simulink model "osek_asap2"  (Simulink 6.0)
settings: Solver=FixedStepDiscrete  StartTime=0.0  StopTime=100.0  RelTol=1e-3
PreLoadFcn:
  | mysig = ASAP2.Signal;
  | mysig.RTWInfo.StorageClass = 'ExportedGlobal';
  | mysig.set('LongID_ASAP2',...
  |   'ExportedGlobal signal - unstructured data',...
  |   'PhysicalMin_ASAP2', -3, ...
  |   'PhysicalMax_ASAP2',  3, ...
  |   'Units_ASAP2',  'rpm');
  | mysig
  | myprm = ASAP2.Parameter;
  | myprm.RTWInfo.StorageClass = 'ExportedGlobal';
  | myprm.set('LongID_ASAP2',...
  |   'ExportedGlobal parameter - unstructured data',...
  |   'PhysicalMin_ASAP2', 0, ...
  |   'PhysicalMax_ASAP2', 15, ...
  |   'Value', 10, ...
  |   'Units_ASAP2',  'none');
  | myprm
settings Model: Creator=jcarrick  LastModifiedBy=jcarrick  ProdHWDeviceType=Motorola PowerPC
settings SolverCC: PositivePriorityOrder=on
settings DataIOCC: SaveOutput=off  SaveTime=off  SignalLoggingName=sigsOut
settings OptimizationCC: InlineParams=on  OptimizeModelRefInitCode=on  LifeSpan=1
settings DebuggingCC: CheckExecutionContextPreStartOutputMsg=on  CheckExecutionContextRuntimeOutputMsg=on  SolverPrmCheckMsg=none
settings HardwareCC: ProdEndianess=BigEndian  ProdHWDeviceType=Motorola PowerPC
settings RTWCC: SystemTargetFile=osekworks.tlc  GenCodeOnly=on  TemplateMakefile=osek_default_tmf  GenerateReport=on  ProcessScript=osekworks_make_rtw_hook  IncludeHyperlinkInReport=on  LaunchReport=on
settings CodeAppCC: IgnoreCustomStorageClasses=off
settings STFCustomTargetCC: TargetFcnLib=ansi_tfl_tmw.mat  GenFloatMathFcnCalls=ANSI_C  ModelReferenceCompliant=off  CombineOutputUpdateFcns=on  SuppressErrorStatus=on  ERTCustomFileBanners=on  SystemTargetFile=osekworks.tlc  ForcedBaseTarget=off
settings ERTTargetCC: TargetFcnLib=ansi_tfl_tmw.mat  GenFloatMathFcnCalls=ANSI_C  ModelReferenceCompliant=off  SuppressErrorStatus=on  SupportContinuousTime=on  SupportNonInlinedSFcns=on  GenerateASAP2=on  RootIOFormat=Individual Arguments  ERTCustomFileTemplate=osek_file_process.tlc  InitialValueSource=Model
settings CustomProperty: DataType=RTWOptions_EnumType__toolbox_rtw_targets_osek_osek_osekworks_bspName  Value=phycore555
settings EnumStrPairs: String=axiomcmd565
settings SFSimCC: SFSimApplyToAllLibs=on  SFSimBuildMode=Incremental

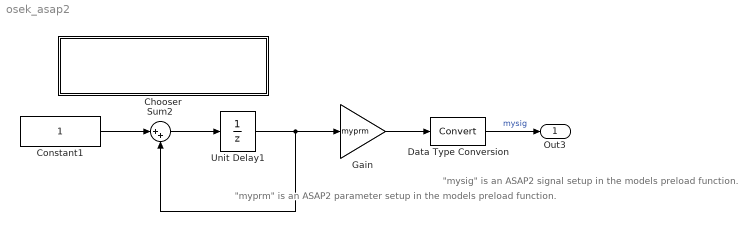
== system osek_asap2 ==
  note: "mysig" is an ASAP2 signal setup
      |  in the models preload function.
  note: "myprm" is an ASAP2 parameter setup
      |  in the models preload function.
  Chooser : Subsystem  LoadFcn=|  PropExecContextAcrossSSBoundary=on  mask{stf=osekworks.tlc}
      | x = osek.prefs.load('osek');                               
      | Implementation = lower(x.Implementation);                  
      | clear x;                                                   
      | switch Implementation                                      
      |  case {'proosek','osekworks'}                              
      |   osek_choose_imp([Implementation,'.tlc']);                
      |   set_param(gcb,'MaskValueString',[Implementation,'.tlc']);
      |  otherwise                                                 
      |   error(['Unrecognized implementation: ' Implementation]); 
      | end                                                        
      | clear Implementation;
      mask prompts: stf "Implementation"
      mask help: Choose OSEK System Target File
      mask init:
      | osek_choose_imp(stf)
      mask StyleString: popup(osekworks.tlc|proosek.tlc)
      mask Display: disp(['Choose System Target File:\nCurrently set to "' strtok(get_param(gcs,'rtwsystemtargetfile')) '"'])
  Constant1 : Constant  OutDataTypeMode=double
  Data Type Conversion : DataTypeConversion  OutDataTypeMode=int32  SaturateOnIntegerOverflow=on  RndMeth=Zero
  Gain : Gain  Gain=myprm  SaturateOnIntegerOverflow=on
  Sum2 : Sum  Inputs=|++  SaturateOnIntegerOverflow=on
  Unit Delay1 : UnitDelay  SampleTime=0.01
  Out3 : Outport
  wires:
  Gain/1 -> Data Type Conversion/1
  Data Type Conversion/1 -> Out3/1  "mysig"
  Unit Delay1/1 -> Sum2/2, Gain/1
  Sum2/1 -> Unit Delay1/1
  Constant1/1 -> Sum2/1

== system osek_asap2/Chooser ==
